simulink model "SailingYachtModel"  (R2012b)
settings: Solver=ode3  StartTime=0.0  StopTime=70  FixedStep=0.05  RelTol=1e-3
undefined symbols (not defined in the file): par
libraries: vrlib x1
settings Model: Creator=Administrator  LastModifiedBy=Dan
settings DataIOCC: SignalLoggingSaveFormat=ModelDataLogs
settings OptimizationCC: InitFltsAndDblsToZero=on
settings DebuggingCC: SaveWithParameterizedLinksMsg=none  SignalResolutionControl=TryResolveAllWithWarning  MultiTaskDSMMsg=warning  MultiTaskCondExecSysMsg=none  FcnCallInpInsideContextMsg=UseLocalSettings  StrictBusMsg=None
settings RTWCC: IncludeERTFirstTime=on
settings CodeAppCC: CustomSymbolStrType=$N$R$M_T  InternalIdentifier=Shortened
settings GRTTargetCC: TargetFcnLib=ansi_tfl_tmw.mat  CombineOutputUpdateFcns=off  GRTInterface=on

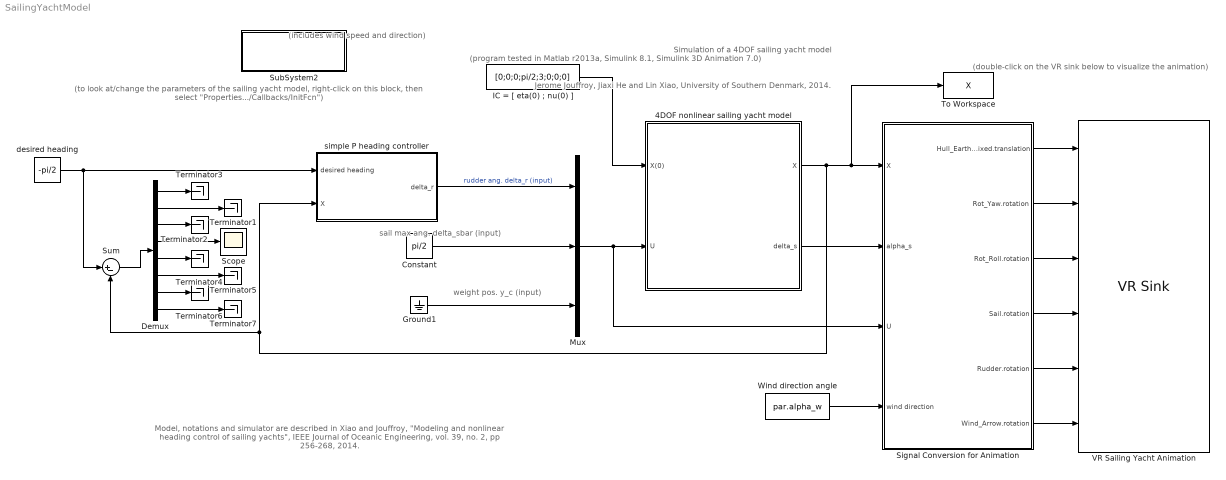
== system SailingYachtModel ==
  note: (includes wind speed and direction)
  note: (program tested in Matlab r2013a, Simulink 8.1, Simulink 3D Animation 7.0)
  note: (double-click on the VR sink below
      | to visualize the animation)
  note: Jerome Jouffroy, Jiaxi He and Lin Xiao,
      | University of Southern Denmark, 2014.
  note: Model, notations and simulator are described in Xiao and Jouffroy, "Modeling and nonlinear heading control of sailing yachts",
      | IEEE Journal of Oceanic Engineering, vol. 39, no. 2, pp 256-268, 2014.
  note: (to look at/change the parameters of the sailing yacht
      | model, right-click on this block, then select
      | "Properties.../Callbacks/InitFcn")
  note: weight pos. y_c (input)
  note: sail max ang. delta_sbar (input)
  note: Simulation of a 4DOF sailing yacht model
  4DOF nonlinear sailing yacht model : Subsystem
  Constant : Constant  Value=pi/2
  Demux : Demux  Outputs=8
  Ground1 : Ground
  IC = [ eta(0) ; nu(0) ] : Constant  Value=[0;0;0;pi/2;3;0;0;0]
  Mux : Mux  Inputs=3
  Scope : Scope
      settings: SaveName=ScopeData2
  Signal Conversion for Animation : Subsystem
  SubSystem2 : Subsystem  InitFcn=|
      | global par
      | par.m = 25900;                         % (kg),mass of the vehicle
      | par.Ixx = 133690;          
      | par.Izz = 24760;      
      | par.Ixz = 2180;                        % moment of inertia
      | par.a11 = 970;   
      | par.a22 = 17430; 
      | par.a44 = 106500;
      | par.a66 = 101650;
      | par.a24 = -13160;
      | par.a26 = -6190; 
      | par.a46 = 4730;                        % (kg),added mass coef.
      | 
      | par.vt = 10;                           % the norm of wind velocity
      | par.alpha_w = pi;                      % the direction of wind (coming from the north, ie going south)
      | 
      | par.rho_a = 1.2;                       % (kg/m^3), air density
      | par.As = 170;                          % (m^2), sail area
      | par.h0 = 0.0005;                       % (m), roughness height
      | par.h1 = 11.58;                        % (m), reference height
      | par.z_s = -11.58;                      % (m), (x,y,z) is the CoE
      | par.xs = 0;
      | par.ys = 0;
      | par.zs = -11.58;                       % (m), (x,y,z) is the CoE
      | par.Xce = 0.6;                         % (m), distance along the mast to the CoE
      | par.Xm = 0.3;                          % (m), x-coordinate of the mast 
      | 
      | par.rho_w = 1025;                      % (kg/m^3), water density
      | par.Ar = 1.17;                         % (m^2), rudder area
      | par.d_r = 1.9;                         % rudder draft
      | par.zeta_r = 0.8;                      % rudder efficiency
      | par.x_r = -8.2;
      | par.z_r = -0.78;                       % (m), (x,y,z) is the CoE
      | par.xr = -8.2;
      | par.yr = 0;
      | par.zr = -0.78;                        % (m), (x,y,z) is the CoE
      | 
      | par.Ak = 8.7;                          % (m^2), keel area
      | par.d_k = 2.49;                        % keel draft
      | par.zeta_k = 0.7;                      % keel efficiency
      | par.x_k = 0;
      | par.z_k = -0.58;                       % (m), (x,y,z) is the CoE
      | par.xk = 0;
      | par.yk = 0;
      | par.zk = -0.58;                        % (m), (x,y,z) is the CoE
      | 
      | par.x_h = 0;
      | par.z_h = -1.18;                       % (m), (x,y,z) is the CoE
      | par.xh = 0;
      | par.yh = 0;
      | par.zh = -1.18;                        % (m), (x,y,z) is the CoE
      | 
      | par.w_c = 60000;                       % (N), crew weight 20000
      | par.x_c = -8;                          % (m), crew position
      | par.y_bm = 3.6;                        % (m), yacht beam
      | 
      | par.a = -5.89;
      | par.b = 8160;
      | par.c = 120000;
      | par.d = 50000;
      mask Display: disp('Parameter Initialization')
  Sum : Sum  Inputs=|+-
  Terminator{1..7} (7 alike) : Terminator
  To Workspace : ToWorkspace  VariableName=X  SampleTime=-1  SaveFormat=Structure With Time
  VR Sailing Yacht Animation : vrlib/VR Sink  InstantiateOnLoad=on  SampleTime=-1  ViewEnable=on  RemoteChange=off  RemoteView=off  FieldsWritten=Hull_EarthFixed.translation.3.1.1.double#Rot_Yaw.rotation.4.1.1.double#Rot_Roll.rotation.4.1.1.double#Sail.rotation.4.1.1.double#Rudder.rotation.4.1.1.double#Wind_Arrow.rotation.4.1.1.double  WorldFileName=SailingYachtAnimation.wrl  WorldDescription=Sailing Yacht VR animation  AutoView=on  VideoDimensions=[]  AllowVariableSize=off  FigureProperties="{'Position', 'Name', 'Viewpoint', 'CameraBound', 'CameraDirection', 'CameraPosition', 'CameraUpVector', 'ZoomFactor', 'Antialiasing', 'Headlight', 'Lighting', 'NavPanel', 'StatusBar', 'ToolBar', 'Textures', 'Transparency', 'Triad', 'Wireframe', 'NavZones', 'NavMode', 'NavSpeed', 'CaptureFileFormat', 'CaptureFileName', 'Record2DCompressMethod', 'Record2DCompressQuality', 'Record2D', 'Record2DFileName', 'Record2DFPS'; [5.0000000000000000e+00   9.2000000000000000e+01   5.7600000000000000e+02   3.8000000000000000e+02], 'Sailing Yacht VR animation', 'overview', 'on', [0.0000000000000000e+00   0.0000000000000000e+00  -1.0000000000000000e+00], [0.0000000000000000e+00   0.0000000000000000e+00   0.0000000000000000e+00], [0.0000000000000000e+00   1.0000000000000000e+00   0.0000000000000000e+00], [1.0000000000000000e+00], 'on', 'on', 'on', 'halfbar', 'on', 'on', 'on', 'on', 'none', 'off', 'off', 'fly', 'normal', 'tif', '%f_anim_%n.tif', 'auto', [7.5000000000000000e+01], 'off', '%f_anim_%n.avi', [1.5000000000000000e+01]}"
  Wind direction angle : Constant  Value=par.alpha_w
  desired heading : Constant  Value=-pi/2
  simple P heading controller : Subsystem
  wires:
  Constant/1 -> Mux/2
  IC = [ eta(0) ; nu(0) ]/1 -> 4DOF nonlinear sailing yacht model/1(X(0))
  Mux/1 -> Signal Conversion for Animation/3(U), 4DOF nonlinear sailing yacht model/2(U)
  4DOF nonlinear sailing yacht model/1(X) -> Signal Conversion for Animation/1(X), To Workspace/1, Sum/2, simple P heading controller/2(X)
  simple P heading controller/1(delta_r) -> Mux/1  "rudder ang. delta_r (input)"
  Ground1/1 -> Mux/3
  desired heading/1 -> Sum/1, simple P heading controller/1(desired heading)
  4DOF nonlinear sailing yacht model/2(delta_s) -> Signal Conversion for Animation/2(alpha_s)
  Wind direction angle/1 -> Signal Conversion for Animation/4(wind direction)
  Signal Conversion for Animation/1(Hull_EarthFixed.translation) -> VR Sailing Yacht Animation/1
  Signal Conversion for Animation/2(Rot_Yaw.rotation) -> VR Sailing Yacht Animation/2
  Signal Conversion for Animation/4(Sail.rotation) -> VR Sailing Yacht Animation/4
  Signal Conversion for Animation/3(Rot_Roll.rotation) -> VR Sailing Yacht Animation/3
  Signal Conversion for Animation/5(Rudder.rotation) -> VR Sailing Yacht Animation/5
  Signal Conversion for Animation/6(Wind_Arrow.rotation) -> VR Sailing Yacht Animation/6
  Sum/1 -> Demux/1
  Demux/4 -> Scope/1
  Demux/1 -> Terminator3/1
  Demux/2 -> Terminator1/1
  Demux/3 -> Terminator2/1
  Demux/5 -> Terminator4/1
  Demux/6 -> Terminator5/1
  Demux/7 -> Terminator6/1
  Demux/8 -> Terminator7/1

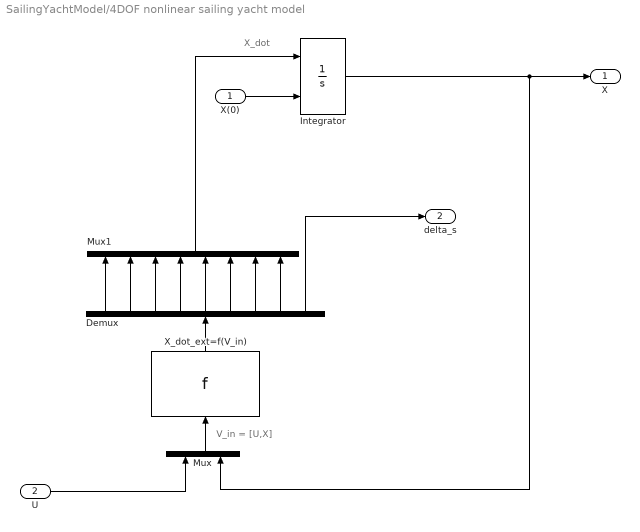
== system SailingYachtModel/4DOF nonlinear sailing yacht model ==
  note: X_dot
  note: V_in = [U,X]
  X(0) : Inport
  U : Inport  Port=2
  Demux : Demux  Outputs=9
  Integrator : Integrator  InitialConditionSource=external  InitialCondition=[0;0;0;pi;1;0;0;0]
  Mux : Mux  Inputs=2
  Mux1 : Mux  Inputs=8
  X_dot_ext=f(V_in) : MATLABFcn  MATLABFcn=f  OutputDimensions=9
  X : Outport
  delta_s : Outport  Port=2
  wires:
  X(0)/1 -> Integrator/2
  Mux/1 -> X_dot_ext=f(V_in)/1
  U/1 -> Mux/1
  Integrator/1 -> X/1, Mux/2
  X_dot_ext=f(V_in)/1 -> Demux/1
  Demux/9 -> delta_s/1
  Demux/8 -> Mux1/8
  Demux/7 -> Mux1/7
  Demux/6 -> Mux1/6
  Demux/5 -> Mux1/5
  Demux/4 -> Mux1/4
  Demux/3 -> Mux1/3
  Demux/2 -> Mux1/2
  Demux/1 -> Mux1/1
  Mux1/1 -> Integrator/1

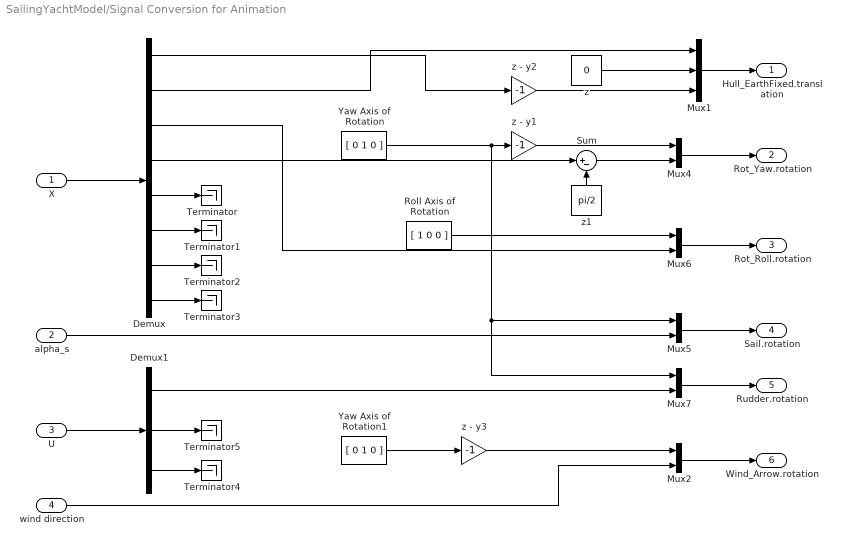
== system SailingYachtModel/Signal Conversion for Animation ==
  X : Inport
  alpha_s : Inport  Port=2
  U : Inport  Port=3
  wind direction : Inport  Port=4
  Demux : Demux  Outputs=8
  Demux1 : Demux  Outputs=3
  Mux1 : Mux  Inputs=3
  Mux{2,4..7} (5 alike) : Mux  Inputs=2
  Roll Axis of Rotation : Constant  Value=[ 1 0 0 ]
  Sum : Sum  Inputs=|+-  SaturateOnIntegerOverflow=on
  Terminator{,1..5} (6 alike) : Terminator
  Yaw Axis of Rotation : Constant  Value=[ 0 1 0 ]
  Yaw Axis of Rotation1 : Constant  Value=[ 0 1 0 ]
  z : Constant  Value=0
  z - y1 : Gain  Gain=-1
  z - y2 : Gain  Gain=-1
  z - y3 : Gain  Gain=-1
  z1 : Constant  Value=pi/2
  Hull_EarthFixed.translation : Outport
  Rot_Yaw.rotation : Outport  Port=2
  Rot_Roll.rotation : Outport  Port=3
  Sail.rotation : Outport  Port=4
  Rudder.rotation : Outport  Port=5
  Wind_Arrow.rotation : Outport  Port=6
  wires:
  Demux/4 -> Sum/1
  Yaw Axis of Rotation/1 -> Mux5/1, Mux7/1, z - y1/1
  Sum/1 -> Mux4/2
  Roll Axis of Rotation/1 -> Mux6/1
  Demux/3 -> Mux6/2
  alpha_s/1 -> Mux5/2
  Demux/1 -> z - y2/1
  z - y2/1 -> Mux1/3
  Demux/2 -> Mux1/1
  z/1 -> Mux1/2
  z - y1/1 -> Mux4/1
  z1/1 -> Sum/2
  Mux1/1 -> Hull_EarthFixed.translation/1
  Demux/5 -> Terminator/1
  Demux/6 -> Terminator1/1
  Demux/7 -> Terminator2/1
  Demux/8 -> Terminator3/1
  X/1 -> Demux/1
  Demux1/3 -> Terminator4/1
  Demux1/2 -> Terminator5/1
  U/1 -> Demux1/1
  Demux1/1 -> Mux7/2
  Mux7/1 -> Rudder.rotation/1
  Mux5/1 -> Sail.rotation/1
  Mux4/1 -> Rot_Yaw.rotation/1
  Yaw Axis of Rotation1/1 -> z - y3/1
  z - y3/1 -> Mux2/1
  wind direction/1 -> Mux2/2
  Mux2/1 -> Wind_Arrow.rotation/1
  Mux6/1 -> Rot_Roll.rotation/1

== system SailingYachtModel/SubSystem2 ==

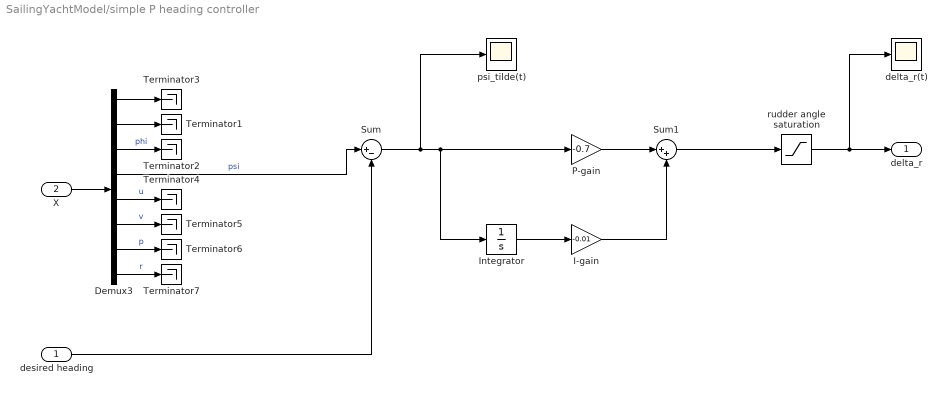
== system SailingYachtModel/simple P heading controller ==
  desired heading : Inport
  X : Inport  Port=2
  Demux3 : Demux  Outputs=8
  I-gain : Gain  Gain=-0.01
  Integrator : Integrator
  P-gain : Gain  Gain=-0.7
  Sum : Sum  Inputs=|+-  SaturateOnIntegerOverflow=on
  Sum1 : Sum  Inputs=|++
  Terminator{1..7} (7 alike) : Terminator
  delta_r(t) : Scope
      settings: YMin=-1.1  YMax=0
  psi_tilde(t) : Scope
      settings: YMin=5.55112e-17  YMax=1.6
  rudder angle saturation : Saturate  UpperLimit=pi/3  LowerLimit=-pi/3  LinearizeAsGain=off
  delta_r : Outport
  wires:
  Demux3/4 -> Sum/1  "psi"
  X/1 -> Demux3/1
  Demux3/1 -> Terminator3/1
  Demux3/2 -> Terminator1/1
  Demux3/3 -> Terminator2/1  "phi"
  Demux3/5 -> Terminator4/1  "u"
  Demux3/6 -> Terminator5/1  "v"
  Demux3/7 -> Terminator6/1  "p"
  Demux3/8 -> Terminator7/1  "r"
  Sum/1 -> psi_tilde(t)/1, Integrator/1, P-gain/1
  P-gain/1 -> Sum1/1
  rudder angle saturation/1 -> delta_r(t)/1, delta_r/1
  desired heading/1 -> Sum/2
  Sum1/1 -> rudder angle saturation/1
  I-gain/1 -> Sum1/2
  Integrator/1 -> I-gain/1
